simulink model "HAdder"  (R2018b)
settings: Solver=VariableStepAuto  StartTime=0.0  StopTime=10.0  RelTol=1e-3
settings Model: Creator=mllax8  LastModifiedBy=mllax8

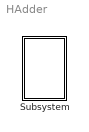
== system HAdder ==
  Subsystem : Subsystem

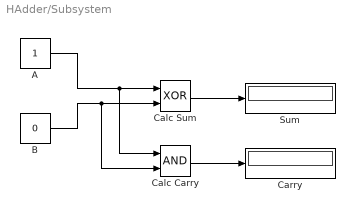
== system HAdder/Subsystem ==
  A : Constant  OutDataTypeStr=boolean
  B : Constant  Value=0  OutDataTypeStr=boolean
  Calc Carry : Logic  AllPortsSameDT=off  OutDataTypeStr=boolean
  Calc Sum : Logic  Operator=XOR  AllPortsSameDT=off  OutDataTypeStr=boolean
  Carry : Display
  Sum : Display
  wires:
  B/1 -> Calc Carry/2, Calc Sum/2
  Calc Carry/1 -> Carry/1
  Calc Sum/1 -> Sum/1
  A/1 -> Calc Carry/1, Calc Sum/1
